simulink model "xaui"  (Simulink 7.3)
settings: Solver=ode45  StartTime=0.0  StopTime=10.0  RelTol=1e-3
undefined symbols (not defined in the file or in its folder): ROACH
libraries: xbsIndex_r4 x21, xps_library x11
settings Model: Creator=rprimian  LastModifiedBy=rprimian

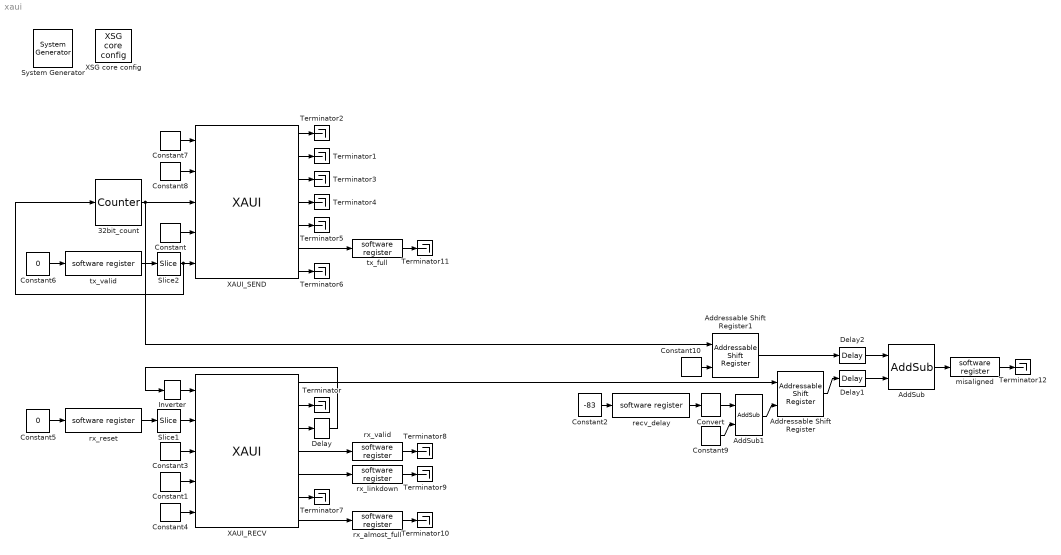
== system xaui ==
  " System Generator" : xbsIndex_r4/ System Generator  Tag=genX  SystemSampleTime=-1  xilinxfamily=virtex5  part=xc5vsx95t  speed=-1  package=ff1136  synthesis_tool=XST  clock_wrapper=Clock Enables  directory=./xaui/sysgen  testbench=off  simulink_period=1  sysclk_period=5  dcm_input_clock_period=100  incr_netlist=off  trim_vbits=Everywhere in SubSystem  dbl_ovrd=According to Block Masks  core_generation=According to Block Masks  run_coregen=off  deprecated_control=off  eval_field=0  block_type=sysgen
      settings: block_version=11.3
  32bit_count : xbsIndex_r4/Counter  cnt_type=Free Running  cnt_to=Inf  operation=Up  start_count=0  cnt_by_val=1  arith_type=Unsigned  n_bits=32  bin_pt=0  load_pin=off  rst=off  en=on  explicit_period=on  period=1  dbl_ovrd=off  use_behavioral_HDL=off  implementation=Fabric  block_type=counter
      settings: block_version=11.3
  AddSub : xbsIndex_r4/AddSub  mode=Subtraction  use_carryin=off  use_carryout=off  en=off  latency=3  precision=Full  arith_type=Unsigned  n_bits=16  bin_pt=14  quantization=Truncate  overflow=Wrap  dbl_ovrd=off  use_behavioral_HDL=off  hw_selection=Fabric  pipelined=on  block_type=addsub
      settings: block_version=11.3
  AddSub1 : xbsIndex_r4/AddSub  mode=Addition  use_carryin=off  use_carryout=off  en=off  latency=2  precision=User Defined  arith_type=Unsigned  n_bits=9  bin_pt=0  quantization=Truncate  overflow=Wrap  dbl_ovrd=off  use_behavioral_HDL=off  hw_selection=Fabric  pipelined=on  block_type=addsub
      settings: block_version=11.3
  Addressable Shift Register : xbsIndex_r4/Addressable Shift Register  infer_latency=on  depth=512  initVector=[0]  en=off  dbl_ovrd=off  use_behavioral_HDL=off  block_type=addrsr
      settings: infoedit="Delay of configurable length.  Any element in the delay line can be addressed and driven onto the output port.<br><br>Hardware notes: This block is implemented using SRL16s. If Virtex-4 or Spartan-3 device is used, multiple SRLC16s are cascaded together."  block_version=11.3
  Addressable Shift Register1 : xbsIndex_r4/Addressable Shift Register  infer_latency=on  depth=512  initVector=[0]  en=off  dbl_ovrd=off  use_behavioral_HDL=off  block_type=addrsr
      settings: infoedit="Delay of configurable length.  Any element in the delay line can be addressed and driven onto the output port.<br><br>Hardware notes: This block is implemented using SRL16s. If Virtex-4 or Spartan-3 device is used, multiple SRLC16s are cascaded together."  block_version=11.3
  Constant : xbsIndex_r4/Constant  arith_type=Unsigned  const=0  n_bits=4  bin_pt=0  explicit_period=on  period=1  equ=P=C  opselect=C  inp2=PCIN>>17  opr=+  inp1=P  carry=CIN  dbl_ovrd=off  block_type=constant
      settings: block_version=11.3
  Constant1 : xbsIndex_r4/Constant  arith_type=Unsigned  const=0  n_bits=4  bin_pt=0  explicit_period=on  period=1  equ=P=C  opselect=C  inp2=PCIN>>17  opr=+  inp1=P  carry=CIN  dbl_ovrd=off  block_type=constant
      settings: block_version=11.3
  Constant10 : xbsIndex_r4/Constant  arith_type=Unsigned  const=2^8 - 1  n_bits=8  bin_pt=0  explicit_period=off  period=1  equ=P=C  opselect=C  inp2=PCIN>>17  opr=+  inp1=P  carry=CIN  dbl_ovrd=off  block_type=constant
      settings: block_version=11.3
  Constant2 : Constant  Value=-83  OutDataType=fixdt(1, 16)  OutScaling=2^0
  Constant3 : xbsIndex_r4/Constant  arith_type=Unsigned  const=0  n_bits=32  bin_pt=0  explicit_period=on  period=1  equ=P=C  opselect=C  inp2=PCIN>>17  opr=+  inp1=P  carry=CIN  dbl_ovrd=off  block_type=constant
      settings: block_version=11.3
  Constant4 : xbsIndex_r4/Constant  arith_type=Boolean  const=0  n_bits=32  bin_pt=0  explicit_period=on  period=1  equ=P=C  opselect=C  inp2=PCIN>>17  opr=+  inp1=P  carry=CIN  dbl_ovrd=off  block_type=constant
      settings: block_version=11.3
  Constant5 : Constant  Value=0  OutDataType=fixdt(1, 16)  OutScaling=2^0
  Constant6 : Constant  Value=0  OutDataType=fixdt(1, 16)  OutScaling=2^0
  Constant7 : xbsIndex_r4/Constant  arith_type=Boolean  const=0  n_bits=32  bin_pt=0  explicit_period=on  period=1  equ=P=C  opselect=C  inp2=PCIN>>17  opr=+  inp1=P  carry=CIN  dbl_ovrd=off  block_type=constant
      settings: block_version=11.3
  Constant8 : xbsIndex_r4/Constant  arith_type=Boolean  const=0  n_bits=32  bin_pt=0  explicit_period=on  period=1  equ=P=C  opselect=C  inp2=PCIN>>17  opr=+  inp1=P  carry=CIN  dbl_ovrd=off  block_type=constant
      settings: block_version=11.3
  Constant9 : xbsIndex_r4/Constant  arith_type=Unsigned  const=2^8 - 1  n_bits=8  bin_pt=0  explicit_period=off  period=1  equ=P=C  opselect=C  inp2=PCIN>>17  opr=+  inp1=P  carry=CIN  dbl_ovrd=off  block_type=constant
      settings: block_version=11.3
  Convert : xbsIndex_r4/Convert  arith_type="Signed  (2's comp)"  n_bits=8  bin_pt=0  quantization=Truncate  overflow=Wrap  latency=2  dbl_ovrd=off  pipeline=on  block_type=convert
      settings: block_version=11.3
  Delay : xbsIndex_r4/Delay  en=off  latency=32  dbl_ovrd=off  reg_retiming=off  block_type=delay
      settings: block_version=11.3
  Delay1 : xbsIndex_r4/Delay  en=off  latency=5  dbl_ovrd=off  reg_retiming=off  block_type=delay
      settings: block_version=11.3
  Delay2 : xbsIndex_r4/Delay  en=off  latency=5  dbl_ovrd=off  reg_retiming=off  block_type=delay
      settings: block_version=11.3
  Inverter : xbsIndex_r4/Inverter  en=off  latency=0  dbl_ovrd=off  block_type=inv
      settings: block_version=11.3
  Slice1 : xbsIndex_r4/Slice  nbits=9  boolean_output=on  mode=Lower Bit Location + Width  bit1=0  base1=MSB of Input  bit0=0  base0=LSB of Input  dbl_ovrd=off  block_type=slice
      settings: block_version=11.3
  Slice2 : xbsIndex_r4/Slice  nbits=9  boolean_output=on  mode=Lower Bit Location + Width  bit1=0  base1=MSB of Input  bit0=0  base0=LSB of Input  dbl_ovrd=off  block_type=slice
      settings: block_version=11.3
  Terminator{,1..12} (13 alike) : Terminator
  XAUI_RECV : xps_library/XAUI  Tag=xps:xaui  SystemSampleTime=-1  demux=2  port=ROACH:1  open_phy=off  show_param=off  pre_emph=3  swing=800
  XAUI_SEND : xps_library/XAUI  Tag=xps:xaui  SystemSampleTime=-1  demux=2  port=ROACH:0  open_phy=off  show_param=off  pre_emph=3  swing=800
  XSG core config : xps_library/XSG core config  Tag=xps:xsg  SystemSampleTime=-1  hw_sys=ROACH:sx95t  ibob_linux=off  clk_src=sys_clk2x  iBOB_clk_src=sys_clk  BEE2_ctrl_clk_src=sys_clk  BEE2_usr_clk_src=sys_clk  ROACH_clk_src=sys_clk2x  CORR_clk_src=sys_clk  gpio_clk_io_group=iBOB:sma  gpio_clk_bit_index=0  clk_rate=200  sample_period=1  synthesis_tool=XST  mpc_type=powerpc440_ext
  misaligned : xps_library/software register  Tag=xps:sw_reg  SystemSampleTime=-1  io_dir=To Processor  arith_type="Signed  (2's comp)"  bitwidth=32  bin_pt=0  sample_period=1  gw_name=xaui_misaligned_user_data_in
  recv_delay : xps_library/software register  Tag=xps:sw_reg  SystemSampleTime=-1  io_dir=From Processor  arith_type="Signed  (2's comp)"  bitwidth=32  bin_pt=0  sample_period=1  gw_name=xaui_recv_delay_user_data_out
  rx_almost_full : xps_library/software register  Tag=xps:sw_reg  SystemSampleTime=-1  io_dir=To Processor  arith_type=Unsigned  bitwidth=32  bin_pt=0  sample_period=1  gw_name=xaui_rx_almost_full_user_data_in
  rx_linkdown : xps_library/software register  Tag=xps:sw_reg  SystemSampleTime=-1  io_dir=To Processor  arith_type=Unsigned  bitwidth=32  bin_pt=0  sample_period=1  gw_name=xaui_rx_linkdown_user_data_in
  rx_reset : xps_library/software register  Tag=xps:sw_reg  SystemSampleTime=-1  io_dir=From Processor  arith_type=Unsigned  bitwidth=32  bin_pt=0  sample_period=1  gw_name=xaui_rx_reset_user_data_out
  rx_valid : xps_library/software register  Tag=xps:sw_reg  SystemSampleTime=-1  io_dir=To Processor  arith_type=Unsigned  bitwidth=32  bin_pt=0  sample_period=1  gw_name=xaui_rx_valid_user_data_in
  tx_full : xps_library/software register  Tag=xps:sw_reg  SystemSampleTime=-1  io_dir=To Processor  arith_type=Unsigned  bitwidth=32  bin_pt=0  sample_period=1  gw_name=xaui_tx_full_user_data_in
  tx_valid : xps_library/software register  Tag=xps:sw_reg  SystemSampleTime=-1  io_dir=From Processor  arith_type=Unsigned  bitwidth=32  bin_pt=0  sample_period=1  gw_name=xaui_tx_valid_user_data_out
  wires:
  XAUI_RECV/2 -> Terminator/1
  XAUI_SEND/2 -> Terminator1/1
  Constant/1 -> XAUI_SEND/4
  Constant1/1 -> XAUI_RECV/4
  XAUI_RECV/3 -> Delay/1
  Delay/1 -> Inverter/1
  Inverter/1 -> XAUI_RECV/1
  XAUI_SEND/1 -> Terminator2/1
  XAUI_SEND/3 -> Terminator3/1
  XAUI_SEND/4 -> Terminator4/1
  XAUI_SEND/5 -> Terminator5/1
  XAUI_SEND/7 -> Terminator6/1
  XAUI_RECV/6 -> Terminator7/1
  XAUI_RECV/1 -> Addressable Shift Register/1
  Constant2/1 -> recv_delay/1
  Constant3/1 -> XAUI_RECV/3
  Constant4/1 -> XAUI_RECV/5
  Constant5/1 -> rx_reset/1
  rx_reset/1 -> Slice1/1
  Slice1/1 -> XAUI_RECV/2
  XAUI_RECV/4 -> rx_valid/1
  XAUI_RECV/5 -> rx_linkdown/1
  rx_valid/1 -> Terminator8/1
  rx_linkdown/1 -> Terminator9/1
  rx_almost_full/1 -> Terminator10/1
  XAUI_RECV/7 -> rx_almost_full/1
  32bit_count/1 -> XAUI_SEND/3, Addressable Shift Register1/1
  Constant7/1 -> XAUI_SEND/1
  Constant6/1 -> tx_valid/1
  tx_valid/1 -> Slice2/1
  Slice2/1 -> XAUI_SEND/5, 32bit_count/1
  Constant8/1 -> XAUI_SEND/2
  tx_full/1 -> Terminator11/1
  XAUI_SEND/6 -> tx_full/1
  Addressable Shift Register/1 -> Delay1/1
  misaligned/1 -> Terminator12/1
  AddSub/1 -> misaligned/1
  recv_delay/1 -> Convert/1
  Convert/1 -> AddSub1/1
  AddSub1/1 -> Addressable Shift Register/2
  Constant9/1 -> AddSub1/2
  Constant10/1 -> Addressable Shift Register1/2
  Addressable Shift Register1/1 -> Delay2/1
  Delay1/1 -> AddSub/2
  Delay2/1 -> AddSub/1
